simulink model "question5"  (R2023b)
settings: Solver=VariableStepAuto  StartTime=0.0  StopTime=50  RelTol=1e-3
values from neighbouring files (symbols this model uses):
  A = [-8.8487+(a-b)/5,-0.0399,-5.55+(c+d)/10,3.5846 ... (first row only)    [main_func.m]    (also in question3.m = [-8.8487+(a-b)/5, -0.0399, -5.55+(c+d)/10, 3.5846)
  B = [0.0564+b/(10+c),0.0319 ... (first row only)    [main_func.m]    (also in question3.m = [0.0564+b/(10+c), 0.0319)
  C = [-3.2988,-2.1932+(10*c+d)/(100+5*a),0.037,-0.0109 ... (first row only)    [main_func.m]    (also in question3.m = [-3.2988, -2.1932+(10*c+d)/(100+5*a), 0.037, -0.0109)
undefined symbols (not defined in the file or in its folder): K5, L5
settings Model: Creator=Fan Xiuqi  LastModifiedBy=Fan Xiuqi

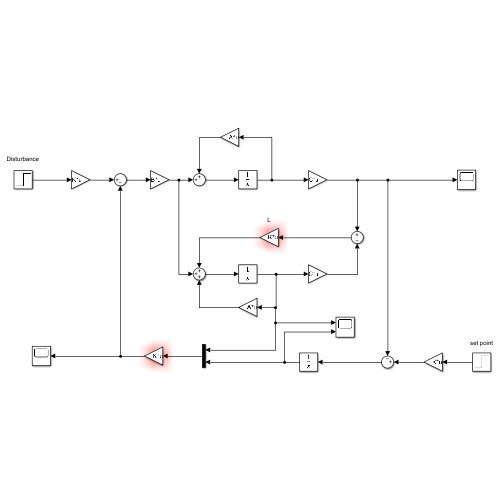
[thumbnail: Simulink's stored preview of the top-level diagram]
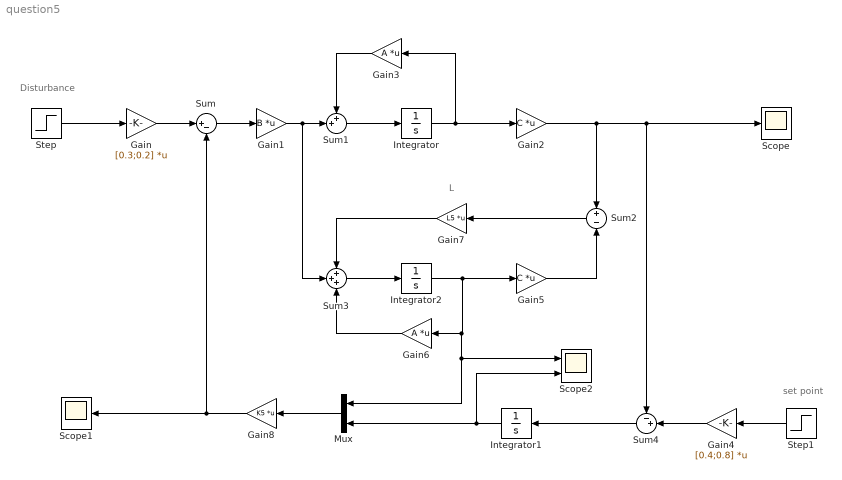
== system question5 ==
  note: L
  note: Disturbance
  note: set point
  Gain : Gain  Gain=[0.3;0.2]  Multiplication=Matrix(K*u)
  Gain1 : Gain  Gain=B  Multiplication=Matrix(K*u)
  Gain2 : Gain  Gain=C  Multiplication=Matrix(K*u)
  Gain3 : Gain  Gain=A  Multiplication=Matrix(K*u)
  Gain4 : Gain  Gain=[0.4;0.8]  Multiplication=Matrix(K*u)
  Gain5 : Gain  Gain=C  Multiplication=Matrix(K*u)
  Gain6 : Gain  Gain=A  Multiplication=Matrix(K*u)
  Gain7 : Gain  Gain=L5  Multiplication=Matrix(K*u)
  Gain8 : Gain  Gain=K5  Multiplication=Matrix(K*u)
  Integrator : Integrator
  Integrator1 : Integrator
  Integrator2 : Integrator
  Mux : Mux  Inputs=2
  Scope : Scope
  Scope1 : Scope
  Scope2 : Scope  NumInputPorts=2
  Step : Step  Time=10  SampleTime=0
  Step1 : Step  SampleTime=0
  Sum : Sum  Inputs=|+-
  Sum1 : Sum  Inputs=++|
  Sum2 : Sum  Inputs=+|-
  Sum3 : Sum  Inputs=+++
  Sum4 : Sum  Inputs=-+|
  wires:
  Gain1/1 -> Sum1/2, Sum3/2
  Sum1/1 -> Integrator/1
  Integrator/1 -> Gain2/1, Gain3/1
  Step1/1 -> Gain4/1
  Integrator1/1 -> Scope2/2, Mux/2
  Gain2/1 -> Scope/1, Sum4/1, Sum2/1
  Gain5/1 -> Sum2/2
  Sum2/1 -> Gain7/1
  Integrator2/1 -> Mux/1, Scope2/1, Gain6/1, Gain5/1
  Sum3/1 -> Integrator2/1
  Gain6/1 -> Sum3/3
  Gain7/1 -> Sum3/1
  Sum/1 -> Gain1/1
  Gain4/1 -> Sum4/2
  Sum4/1 -> Integrator1/1
  Gain8/1 -> Sum/2, Scope1/1
  Mux/1 -> Gain8/1
  Step/1 -> Gain/1
  Gain/1 -> Sum/1
  Gain3/1 -> Sum1/1
